simulink model "Perfect_Lineaer"  (R2017a)
settings: Solver=VariableStepAuto  StartTime=0.0  StopTime=17  FixedStep=0.01  RelTol=1e-3
values from neighbouring files (symbols this model uses):
  A = [-4.65E-06	0.0001701	-0.0002836	0	0	0	-2.56E-06	-7.97E-06	3.61E-06 ... (first row only)    [surfaces_setup_test.m]
  A0 = [-4.65E-06	0.0001701	-0.0002836	0	0	0	0	-1.43	0 ... (first row only)    [surfaces_setup_test.m]
  a0_s2345 = [0;0;0.05;0.05]    [HW5_4_surfaces.m]    (also in TEST_aerosetup.m; surfaces_setup_test.m)
  A_2345 = c_2345.*b_2345    [HW5_4_surfaces.m]    (also in TEST_aerosetup.m; surfaces_setup_test.m)
  Aileron_left = 0    [HW5_4_surfaces.m]    (also in TEST_aerosetup.m; surfaces_setup_test.m)
  Aileron_right = 0    [HW5_4_surfaces.m]    (also in TEST_aerosetup.m; surfaces_setup_test.m)
  B = [-7.98E-09	7.83E-09	1.68E-09	2.75E-10 ... (first row only)    [surfaces_setup_test.m]
  B0 = [-6.2	6.2	0	0.45 ... (first row only)    [surfaces_setup_test.m]
  c_2345 = [0.075;0.08;0.1;0.1]    [HW5_4_surfaces.m]    (also in TEST_aerosetup.m; surfaces_setup_test.m)
  CD0_s2345 = [0.01;0.01;0.01;0.01]    [HW5_4_surfaces.m]    (also in TEST_aerosetup.m; surfaces_setup_test.m)
  CDa_s2345 = [1;1;1;1]    [HW5_4_surfaces.m]    (also in TEST_aerosetup.m; surfaces_setup_test.m)
  CL0_2345 = [0;0; 0.05; 0.05]    [HW5_4_surfaces.m]    (also in TEST_aerosetup.m; surfaces_setup_test.m)
  CLa = 2*pi*(r./(2+r))    [HW5_4_surfaces.m]    (also in TEST_aerosetup.m; surfaces_setup_test.m)
  CM0_s2345 = [0;0;-0.05;-0.05]    [HW5_4_surfaces.m]    (also in TEST_aerosetup.m; surfaces_setup_test.m)
  CMa_s2345 = [0; 0; 0; 0]    [HW5_4_surfaces.m]    (also in TEST_aerosetup.m; surfaces_setup_test.m)
  e_s2345 = [0.8;0.8;0.9;0.9]    [HW5_4_surfaces.m]    (also in TEST_aerosetup.m; surfaces_setup_test.m)
  elevator = 0    [HW5_4_surfaces.m]    (also in TEST_aerosetup.m; surfaces_setup_test.m)
  Fext_N = -g_EN * m    [HW5_4_surfaces.m]    (also in TEST_aerosetup.m = [10 10 10]; surfaces_setup_test.m)
  g_EN = [0; 0; 9.81]    [HW5_4_surfaces.m]    (also in TEST_aerosetup.m = [0; 0; 9.8]; surfaces_setup_test.m)
  i_s2345 = [0; 0; 0.05; 0.05;]    [HW5_4_surfaces.m]    (also in TEST_aerosetup.m; surfaces_setup_test.m)
  J_cgp = ones(3)    [surfaces_setup_test.m]
  M_total = sum(MnG(:,1))/1000    [HW5_4_surfaces.m]    (also in TEST_aerosetup.m; surfaces_setup_test.m = sum(MnG1(:,1))/1000)
  Mext_B = [0; 0; 0]    [HW5_4_surfaces.m]    (also in TEST_aerosetup.m = [1; 1; 1]; surfaces_setup_test.m)
  p_E_BE_ini = p_E_BE_ini_deg .* [deg2rad; deg2rad; 1]    [HW5_4_surfaces.m]    (also in TEST_aerosetup.m; surfaces_setup_test.m)
  r = b_2345./c_2345    [HW5_4_surfaces.m]    (also in TEST_aerosetup.m; surfaces_setup_test.m)
  Rearth = 6371000    [HW5_4_surfaces.m]    (also in TEST_aerosetup.m; surfaces_setup_test.m)
  rudder = 0    [HW5_4_surfaces.m]    (also in TEST_aerosetup.m; surfaces_setup_test.m)
  Theta_ini = Theta_ini_deg * deg2rad    [HW5_4_surfaces.m]    (also in TEST_aerosetup.m; surfaces_setup_test.m)
  U0 = [Aileron_right;Aileron_left;elevator;rudder]    [surfaces_setup_test.m]
  v_N_AE = [0;0;0]    [HW5_4_surfaces.m]    (also in TEST_aerosetup.m; surfaces_setup_test.m)
  Vbbe_int = [10; 0; 0]    [HW5_4_surfaces.m]    (also in TEST_aerosetup.m; surfaces_setup_test.m = [5; 0; 0])
  w_B_BE_ini = [1e0; 1e-2; 1e-2]    [HW5_4_surfaces.m]    (also in TEST_aerosetup.m; surfaces_setup_test.m)
  X0 = [w_B_BE_ini;Theta_ini;Vbbe_int]    [surfaces_setup_test.m]
  xyz_s = [[-0.76 0 0.16];[-0.76 0 -0.09];[-0.23 0.44 0];[-0.23 -0.44 0];]    [HW5_4_surfaces.m]    (also in TEST_aerosetup.m; surfaces_setup_test.m)
undefined symbols (not defined in the file or in its folder): Discrete, Earth, K, Time, WGS84
libraries: simulink x83, aerolibfltsims x5, dspsrcs4 x4, simulink_extras x4, dspinverses x3, vrlib x2, sharedtransform x1, aerolibtransform2 x1, aerolibutil x1, sharedutil x1, ctrlSharedLib x1
(part 5 of 8)

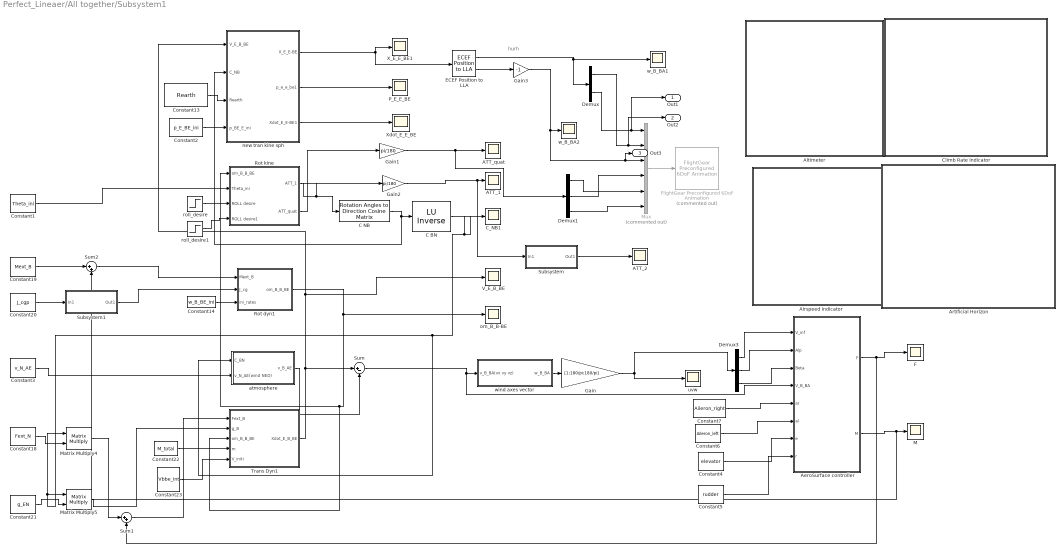
== system Perfect_Lineaer/All together/Subsystem1 ==
  note: hurh
  ATT_1 : Scope
  ATT_2 : Scope
  ATT_quat : Scope
  AeroSurface controller : Subsystem
  Airspeed Indicator : Subsystem  DialogController=aeroblksHMICreateDDGDialog  IsWebBlock=on  mask(MWDashboardBlock){webBlockId=e5e3171d-ff29-4451-bf74-d38876eec561, webBlockType=airspeedindicator, ShowInLibBrowser=on, ShowInitialText=on, HMISrcModelName=Perfect_Lineaer}
      mask prompts: webBlockId "WebBlock Id"; webBlockType "WebBlock Type"; HMISrcModelName "Source Model"
      mask help: aeroblksHMI:aeroblkhmi:AirspeedIndicatorDialogDesc
      mask Help: eval('asbhmihelp(''airspeedindicator'')');
      mask Display:
      | if strcmp(get_param(bdroot(gcb),'BlockDiagramType'), 'library')
      |  image([(matlabroot) '/toolbox/aeroblks/aeroblks/hmi/icons/AirspeedIndicatorIcon.svg'])
      | end
  Altimeter : Subsystem  DialogController=aeroblksHMICreateDDGDialog  IsWebBlock=on  mask(MWDashboardBlock){webBlockId=36990637-e96a-433a-956a-f44ed4ed9d1e, webBlockType=altimeter, ShowInLibBrowser=on, ShowInitialText=on, HMISrcModelName=Perfect_Lineaer}
      mask prompts: webBlockId "WebBlock Id"; webBlockType "WebBlock Type"; HMISrcModelName "Source Model"
      mask help: aeroblksHMI:aeroblkhmi:AltimeterDialogDesc
      mask Help: eval('asbhmihelp(''altimeter'')');
      mask Display:
      | if strcmp(get_param(bdroot(gcb),'BlockDiagramType'), 'library')
      |  image([(matlabroot) '/toolbox/aeroblks/aeroblks/hmi/icons/AltimeterIcon.svg'])
      | end
  Artificial Horizon : Subsystem  DialogController=aeroblksHMICreateDDGDialog  IsWebBlock=on  mask(MWDashboardBlock){webBlockId=4cd5d09c-38f7-433d-892c-50154f5485b8, webBlockType=artificialhorizon, ShowInLibBrowser=on, ShowInitialText=on, HMISrcModelName=Perfect_Lineaer}
      mask prompts: webBlockId "WebBlock Id"; webBlockType "WebBlock Type"; HMISrcModelName "Source Model"
      mask help: aeroblksHMI:aeroblkhmi:ArtificialHorizonDialogDesc
      mask Help: eval('asbhmihelp(''artificialhorizon'')');
      mask Display:
      | if strcmp(get_param(bdroot(gcb),'BlockDiagramType'), 'library')
      |  image([(matlabroot) '/toolbox/aeroblks/aeroblks/hmi/icons/ArtificialHorizonIcon.svg'])
      | end
  C BN : dspinverses/ LU Inverse
      settings: SourceProductName=DSP System Toolbox
  C NB : sharedtransform/Rotation Angles to Direction Cosine Matrix  rotationOrder=ZYX
  C_NB1 : Scope
  Climb Rate Indicator : Subsystem  DialogController=aeroblksHMICreateDDGDialog  IsWebBlock=on  mask(MWDashboardBlock){webBlockId=79e6d40e-4c73-4bf3-981b-23b4e158f69b, webBlockType=climbindicator, ShowInLibBrowser=on, ShowInitialText=on, HMISrcModelName=Perfect_Lineaer}
      mask prompts: webBlockId "WebBlock Id"; webBlockType "WebBlock Type"; HMISrcModelName "Source Model"
      mask help: aeroblksHMI:aeroblkhmi:ClimbIndicatorDialogDesc
      mask Help: eval('asbhmihelp(''climbindicator'')');
      mask Display:
      | if strcmp(get_param(bdroot(gcb),'BlockDiagramType'), 'library')
      |  image([(matlabroot) '/toolbox/aeroblks/aeroblks/hmi/icons/ClimbIndicatorIcon.svg'])
      | end
  Constant1 : Constant  Value=Theta_ini
  Constant13 : Constant  Value=Rearth
  Constant14 : Constant  Value=w_B_BE_ini
  Constant18 : Constant  Value=Fext_N
  Constant19 : Constant  Value=Mext_B
  Constant2 : Constant  Value=p_E_BE_ini  VectorParams1D=off
  Constant20 : Constant  Value=J_cgp
  Constant21 : Constant  Value=g_EN
  Constant22 : Constant  Value=M_total
  Constant23 : Constant  Value=Vbbe_int
  Constant3 : Constant  Value=v_N_AE
  Constant4 : Constant  Value=elevator
  Constant5 : Constant  Value=rudder
  Constant6 : Constant  Value=Aileron_left
  Constant7 : Constant  Value=Aileron_right
  Demux : Demux  Outputs=2
  Demux1 : Demux  Outputs=3
  Demux3 : Demux  Outputs=3
  ECEF Position to LLA : aerolibtransform2/ECEF Position to LLA  units=Metric (MKS)  ptype=Earth (WGS84)  F=1/298.257223563  R=6378137
      settings: SourceProductName=Aerospace Blockset  SourceProductBaseCode=AE
  F : Scope
  FlightGear Preconfigured 6DoF Animation : aerolibfltsims/FlightGear Preconfigured 6DoF Animation  Commented=on  xFlightGearVersion=v3.0  DestinationIpAddress=127.0.0.1  DestinationPort=5502  SampleTime=1/50
      settings: SourceProductName=Aerospace Blockset
  Gain : Gain  Gain=[1;180/pi;180/pi]
  Gain1 : Gain  Gain=pi/180
  Gain2 : Gain  Gain=pi/180
  Gain3 : Gain  Gain=-1
  M : Scope
  Matrix Multiply4 : Product  Multiplication=Matrix(*)
  Matrix Multiply5 : Product  Multiplication=Matrix(*)
  Mux : Mux  Commented=on  Inputs=6
  P_E_E_BE : Scope
  Rot dyn1 : Subsystem
  Rot kine : Subsystem
  Subsystem : Subsystem
  Subsystem1 : Subsystem
  Sum : Sum  Inputs=|+-
  Sum1 : Sum  Inputs=|++
  Sum2 : Sum  Inputs=|++
  Trans Dyn1 : Subsystem
  V_E_B_BE : Scope
  "X_E_E_BE1 " : Scope
  Xdot_E_E_BE : Scope
  atmosphere : Subsystem
  new tran kine sph : Subsystem
  om_B_B-BE : Scope
  roll_desire : Step  Time=0  After=0  SampleTime=0
  roll_desire1 : Step  Time=0  After=0  SampleTime=0
  uvw : Scope
  w_B_BA1 : Scope
  w_B_BA2 : Scope
  wind axes vector : Subsystem
  Out1 : Outport
  Out2 : Outport  Port=2
  Out3 : Outport  Port=3
  wires:
  Subsystem1/1(Out1) -> Rot dyn1/2(J_cg)
  Constant20/1 -> Subsystem1/1(In1)
  Sum1/1 -> Trans Dyn1/1(Fext_B)
  Gain3/1 -> w_B_BA2/1, Out3/1, Mux/3
  ECEF Position to LLA/1 -> Demux/1, w_B_BA1/1
  Constant19/1 -> Sum2/1
  roll_desire/1 -> Rot kine/3(ROLL desire)
  Matrix Multiply4/1 -> Sum1/1
  ECEF Position to LLA/2 -> Gain3/1
  Demux1/2 -> Mux/4
  Gain2/1 -> Subsystem/1(In1), ATT_1/1
  Rot kine/2(ATT_quat) -> Gain1/1
  AeroSurface controller/1(F) -> Sum1/2, F/1
  Demux3/1 -> AeroSurface controller/1(V_inf)
  Demux3/2 -> AeroSurface controller/2(Alp)
  Constant21/1 -> Matrix Multiply5/2
  Demux1/3 -> Mux/6
  C NB/1 -> new tran kine sph/2(C_NB), C BN/1
  Constant5/1 -> AeroSurface controller/8(r)
  Constant7/1 -> AeroSurface controller/5(ar)
  Rot dyn1/1(om_B_B_BE) -> Trans Dyn1/3(om_B_B_BE), Rot kine/1(om_B_B_BE), om_B_B-BE/1
  atmosphere/1(v_B_AE) -> Sum/2
  Sum/1 -> AeroSurface controller/4(V_B_BA), wind axes vector/1(v_B_BA(vx vy vz))
  Constant22/1 -> Trans Dyn1/4(m)
  Constant4/1 -> AeroSurface controller/7(e)
  Constant1/1 -> Rot kine/2(Theta_ini)
  Gain1/1 -> Demux1/1, ATT_quat/1
  Sum2/1 -> Rot dyn1/1(Mext_B)
  AeroSurface controller/2(M) -> Sum2/2, M/1
  Demux1/1 -> Mux/5
  Mux/1 -> FlightGear Preconfigured 6DoF Animation/1
  Constant13/1 -> new tran kine sph/3(Rearth)
  Constant14/1 -> Rot dyn1/3(ini_rates)
  roll_desire1/1 -> Rot kine/4(ROLL desire1)
  new tran kine sph/3(Xdot_E_E-BE1) -> Xdot_E_E_BE/1
  Rot kine/1(ATT_1) -> C NB/1, Gain2/1
  C BN/1 -> atmosphere/1(C_BN), Matrix Multiply5/1, Matrix Multiply4/1, C_NB1/1
  new tran kine sph/1(X_E_E-BE) -> ECEF Position to LLA/1, "X_E_E_BE1 "/1
  Subsystem/1(Out1) -> ATT_2/1
  Constant6/1 -> AeroSurface controller/6(al)
  Constant3/1 -> atmosphere/2(v_N_AE(wind NED))
  new tran kine sph/2(p_e_e_be1) -> P_E_E_BE/1
  Trans Dyn1/1(Xdot_E_B_BE) -> new tran kine sph/1(V_E_B_BE), V_E_B_BE/1, Sum/1
  Gain/1 -> Demux3/1, uvw/1
  Constant18/1 -> Matrix Multiply4/2
  wind axes vector/1(w_B_BA) -> Gain/1
  Constant23/1 -> Trans Dyn1/5(V_initi)
  Demux/1 -> Out2/1, Mux/2
  Demux/2 -> Out1/1, Mux/1
  Demux3/3 -> AeroSurface controller/3(Beta)
  Constant2/1 -> new tran kine sph/4(p_BE_E_ini)
  Matrix Multiply5/1 -> Trans Dyn1/2(g_B)

== system Perfect_Lineaer/All together/Subsystem2 ==
  note: State loop
  note: Inner loop
  Rudder : Inport
  Elevator : Inport  Port=2
  Aileron_left : Inport  Port=3
  A : Gain  Gain=A  Multiplication=Matrix(K*u)
  B : Gain  Gain=B  Multiplication=Matrix(K*u)
  Constant1 : Constant  Value=0
  Constant2 : Constant  Value=X0
  Demux : Demux  Outputs=9
  Integrator : Integrator  InitialConditionSource=external
  KD_Based on Rlocus : Gain
  Mux : Mux  Inputs=9
  Mux1 : Mux
  Scope : Scope
  Scope1 : Scope
  Sum : Sum  Inputs=|++
  Sum1 : Sum  Inputs=|++
  Sum4 : Sum  Inputs=|+-
  selector : Subsystem
  R(yaw) : Outport
  Q(pitch) : Outport  Port=2
  P(roll) : Outport  Port=3
  wires:
  Elevator/1 -> Mux1/3
  Sum1/1 -> Mux/8
  KD_Based on Rlocus/1 -> Sum1/2
  Demux/8 -> Sum1/1
  Rudder/1 -> Mux1/4
  Constant1/1 -> Mux1/1
  Mux1/1 -> B/1
  Mux/1 -> Sum4/1
  Demux/1 -> Mux/1
  Demux/5 -> Mux/5
  A/1 -> Sum/2
  Sum4/1 -> Sum/1
  Integrator/1 -> A/1, selector/1(In1), Scope/1, Sum4/2
  Demux/9 -> Mux/9
  Demux/4 -> Mux/4
  Demux/2 -> Mux/2
  B/1 -> Demux/1
  selector/1(Out1) -> KD_Based on Rlocus/1, Scope1/1
  Sum/1 -> Integrator/1
  Demux/3 -> Mux/3
  Constant2/1 -> Integrator/2
  Demux/6 -> Mux/6
  Demux/7 -> Mux/7
  selector/2(Out2) -> Q(pitch)/1
  selector/3(Out3) -> R(yaw)/1
  selector/4(Out4) -> P(roll)/1
  Aileron_left/1 -> Mux1/2

== system Perfect_Lineaer/All together/Subsystem5 ==
  note: State loop
  note: Inner loop
  Rudder : Inport
  Elevator : Inport  Port=2
  Aileron_left : Inport  Port=3
  A : Gain  Gain=A  Multiplication=Matrix(K*u)
  B : Gain  Gain=B  Multiplication=Matrix(K*u)
  Constant1 : Constant  Value=0
  Constant2 : Constant  Value=X0
  Demux : Demux  Outputs=9
  Integrator : Integrator  InitialConditionSource=external
  KD_Based on Rlocus : Gain
  Mux : Mux  Inputs=9
  Mux1 : Mux
  Scope : Scope
  Scope1 : Scope
  Sum : Sum  Inputs=|++
  Sum1 : Sum  Inputs=|++
  Sum4 : Sum  Inputs=|+-
  selector : Subsystem
  R(yaw) : Outport
  Q(pitch) : Outport  Port=2
  P(roll) : Outport  Port=3
  wires:
  Elevator/1 -> Mux1/3
  Sum1/1 -> Mux/8
  KD_Based on Rlocus/1 -> Sum1/2
  Demux/8 -> Sum1/1
  Rudder/1 -> Mux1/4
  Constant1/1 -> Mux1/1
  Mux1/1 -> B/1
  Mux/1 -> Sum4/1
  Demux/1 -> Mux/1
  Demux/5 -> Mux/5
  A/1 -> Sum/2
  Sum4/1 -> Sum/1
  Integrator/1 -> A/1, selector/1(In1), Scope/1, Sum4/2
  Demux/9 -> Mux/9
  Demux/4 -> Mux/4
  Demux/2 -> Mux/2
  B/1 -> Demux/1
  selector/1(Out1) -> KD_Based on Rlocus/1, Scope1/1
  Sum/1 -> Integrator/1
  Demux/3 -> Mux/3
  Constant2/1 -> Integrator/2
  Demux/6 -> Mux/6
  Demux/7 -> Mux/7
  selector/2(Out2) -> Q(pitch)/1
  selector/3(Out3) -> R(yaw)/1
  selector/4(Out4) -> P(roll)/1
  Aileron_left/1 -> Mux1/2

== system Perfect_Lineaer/All together/Turn Coordinator ==

== system Perfect_Lineaer/Command size/Subsystem ==
  note: State loop
  note: Inner loop
  Rudder : Inport
  A : Gain  Gain=A  Multiplication=Matrix(K*u)
  B : Gain  Gain=B  Multiplication=Matrix(K*u)
  Constant1 : Constant  Value=0
  Constant2 : Constant  Value=X0
  Demux : Demux  Outputs=9
  Integrator : Integrator  InitialConditionSource=external
  KD_Based on Rlocus : Gain
  Mux : Mux  Inputs=9
  Mux1 : Mux
  Scope : Scope
  Scope1 : Scope
  Sum : Sum  Inputs=|++
  Sum1 : Sum  Inputs=|++
  Sum4 : Sum  Inputs=|+-
  selector : Subsystem
  R(yaw) : Outport
  wires:
  Sum1/1 -> Mux/8
  KD_Based on Rlocus/1 -> Sum1/2
  Demux/8 -> Sum1/1
  selector/2(Out2) -> R(yaw)/1
  Rudder/1 -> Mux1/4
  Constant1/1 -> Mux1/1, Mux1/2, Mux1/3
  Mux1/1 -> B/1
  Mux/1 -> Sum4/1
  Demux/1 -> Mux/1
  Demux/5 -> Mux/5
  A/1 -> Sum/2
  Sum4/1 -> Sum/1
  Integrator/1 -> A/1, selector/1(In1), Scope/1, Sum4/2
  Demux/9 -> Mux/9
  Demux/4 -> Mux/4
  Demux/2 -> Mux/2
  B/1 -> Demux/1
  selector/1(Out1) -> KD_Based on Rlocus/1, Scope1/1
  Sum/1 -> Integrator/1
  Demux/3 -> Mux/3
  Constant2/1 -> Integrator/2
  Demux/6 -> Mux/6
  Demux/7 -> Mux/7

== system Perfect_Lineaer/Command size/Subsystem1 ==
  note: State loop
  note: Inner loop
  Elevator : Inport
  A : Gain  Gain=A  Multiplication=Matrix(K*u)
  B : Gain  Gain=B  Multiplication=Matrix(K*u)
  Constant1 : Constant  Value=0
  Constant2 : Constant  Value=X0
  Demux : Demux  Outputs=9
  Integrator : Integrator  InitialConditionSource=external
  KD_Based on Rlocus : Gain
  Mux : Mux  Inputs=9
  Mux1 : Mux
  Scope : Scope
  Scope1 : Scope
  Sum : Sum  Inputs=|++
  Sum1 : Sum  Inputs=|++
  Sum4 : Sum  Inputs=|+-
  selector : Subsystem
  Q(pitch) : Outport
  wires:
  Elevator/1 -> Mux1/3
  Sum1/1 -> Mux/8
  KD_Based on Rlocus/1 -> Sum1/2
  Demux/8 -> Sum1/1
  Constant1/1 -> Mux1/4, Mux1/1, Mux1/2
  Mux1/1 -> B/1
  Mux/1 -> Sum4/1
  Demux/1 -> Mux/1
  Demux/5 -> Mux/5
  A/1 -> Sum/2
  Sum4/1 -> Sum/1
  Integrator/1 -> A/1, Scope/1, Sum4/2, selector/1(In1)
  Demux/9 -> Mux/9
  Demux/4 -> Mux/4
  Demux/2 -> Mux/2
  B/1 -> Demux/1
  selector/1(Out1) -> KD_Based on Rlocus/1, Scope1/1
  Sum/1 -> Integrator/1
  Demux/3 -> Mux/3
  Constant2/1 -> Integrator/2
  Demux/6 -> Mux/6
  Demux/7 -> Mux/7
  selector/2(Out2) -> Q(pitch)/1

== system Perfect_Lineaer/Command size/Subsystem2 ==
  note: State loop
  note: Inner loop
  Rudder : Inport
  A : Gain  Gain=A  Multiplication=Matrix(K*u)
  B : Gain  Gain=B  Multiplication=Matrix(K*u)
  Constant1 : Constant  Value=0
  Constant2 : Constant  Value=X0
  Demux : Demux  Outputs=9
  Integrator : Integrator  InitialConditionSource=external
  KD_Based on Rlocus : Gain
  Mux : Mux  Inputs=9
  Mux1 : Mux
  Scope : Scope
  Scope1 : Scope
  Sum : Sum  Inputs=|++
  Sum1 : Sum  Inputs=|++
  Sum4 : Sum  Inputs=|+-
  selector : Subsystem
  R(yaw) : Outport
  wires:
  Sum1/1 -> Mux/8
  KD_Based on Rlocus/1 -> Sum1/2
  Demux/8 -> Sum1/1
  selector/2(Out2) -> R(yaw)/1
  Rudder/1 -> Mux1/4
  Constant1/1 -> Mux1/1, Mux1/2, Mux1/3
  Mux1/1 -> B/1
  Mux/1 -> Sum4/1
  Demux/1 -> Mux/1
  Demux/5 -> Mux/5
  A/1 -> Sum/2
  Sum4/1 -> Sum/1
  Integrator/1 -> A/1, selector/1(In1), Scope/1, Sum4/2
  Demux/9 -> Mux/9
  Demux/4 -> Mux/4
  Demux/2 -> Mux/2
  B/1 -> Demux/1
  selector/1(Out1) -> KD_Based on Rlocus/1, Scope1/1
  Sum/1 -> Integrator/1
  Demux/3 -> Mux/3
  Constant2/1 -> Integrator/2
  Demux/6 -> Mux/6
  Demux/7 -> Mux/7

== system Perfect_Lineaer/Command size/Subsystem3 ==
  note: State loop
  note: Inner loop
  Elevator : Inport
  A : Gain  Gain=A  Multiplication=Matrix(K*u)
  B : Gain  Gain=B  Multiplication=Matrix(K*u)
  Constant1 : Constant  Value=0
  Constant2 : Constant  Value=X0
  Demux : Demux  Outputs=9
  Integrator : Integrator  InitialConditionSource=external
  KD_Based on Rlocus : Gain
  Mux : Mux  Inputs=9
  Mux1 : Mux
  Scope : Scope
  Scope1 : Scope
  Sum : Sum  Inputs=|++
  Sum1 : Sum  Inputs=|++
  Sum4 : Sum  Inputs=|+-
  selector : Subsystem
  Q(pitch) : Outport
  wires:
  Elevator/1 -> Mux1/3
  Sum1/1 -> Mux/8
  KD_Based on Rlocus/1 -> Sum1/2
  Demux/8 -> Sum1/1
  Constant1/1 -> Mux1/4, Mux1/1, Mux1/2
  Mux1/1 -> B/1
  Mux/1 -> Sum4/1
  Demux/1 -> Mux/1
  Demux/5 -> Mux/5
  A/1 -> Sum/2
  Sum4/1 -> Sum/1
  Integrator/1 -> A/1, Scope/1, Sum4/2, selector/1(In1)
  Demux/9 -> Mux/9
  Demux/4 -> Mux/4
  Demux/2 -> Mux/2
  B/1 -> Demux/1
  selector/1(Out1) -> KD_Based on Rlocus/1, Scope1/1
  Sum/1 -> Integrator/1
  Demux/3 -> Mux/3
  Constant2/1 -> Integrator/2
  Demux/6 -> Mux/6
  Demux/7 -> Mux/7
  selector/2(Out2) -> Q(pitch)/1

== system Perfect_Lineaer/Command size/Subsystem4 ==
  note: State loop
  note: Inner loop
  Aileron_r : Inport
  Aileron_l : Inport  Port=2
  A : Gain  Gain=A  Multiplication=Matrix(K*u)
  B : Gain  Gain=B  Multiplication=Matrix(K*u)
  Constant1 : Constant  Value=0
  Constant2 : Constant  Value=X0
  Demux : Demux  Outputs=9
  Integrator : Integrator  InitialConditionSource=external
  KD_Based on Rlocus : Gain
  Mux : Mux  Inputs=9
  Mux1 : Mux
  Scope : Scope
  Scope1 : Scope
  Sum : Sum  Inputs=|++
  Sum1 : Sum  Inputs=|++
  Sum4 : Sum  Inputs=|+-
  selector : Subsystem
  P(roll) : Outport
  wires:
  Aileron_r/1 -> Mux1/1
  Aileron_l/1 -> Mux1/2
  Sum1/1 -> Mux/8
  KD_Based on Rlocus/1 -> Sum1/2
  Demux/8 -> Sum1/1
  selector/2(Out2) -> P(roll)/1
  Constant1/1 -> Mux1/4, Mux1/3
  Mux1/1 -> B/1
  Mux/1 -> Sum4/1
  Demux/1 -> Mux/1
  Demux/5 -> Mux/5
  A/1 -> Sum/2
  Sum4/1 -> Sum/1
  Integrator/1 -> A/1, selector/1(In1), Scope/1, Sum4/2
  Demux/9 -> Mux/9
  Demux/4 -> Mux/4
  Demux/2 -> Mux/2
  B/1 -> Demux/1
  selector/1(Out1) -> KD_Based on Rlocus/1, Scope1/1
  Sum/1 -> Integrator/1
  Demux/3 -> Mux/3
  Constant2/1 -> Integrator/2
  Demux/6 -> Mux/6
  Demux/7 -> Mux/7

== system Perfect_Lineaer/Command size/Subsystem9 ==
  note: State loop
  note: Inner loop
  Aileron_r : Inport
  Aileron_l : Inport  Port=2
  A : Gain  Gain=A  Multiplication=Matrix(K*u)
  B : Gain  Gain=B  Multiplication=Matrix(K*u)
  Constant1 : Constant  Value=0
  Constant2 : Constant  Value=X0
  Demux : Demux  Outputs=9
  Integrator : Integrator  InitialConditionSource=external
  KD_Based on Rlocus : Gain
  Mux : Mux  Inputs=9
  Mux1 : Mux
  Scope : Scope
  Scope1 : Scope
  Sum : Sum  Inputs=|++
  Sum1 : Sum  Inputs=|++
  Sum4 : Sum  Inputs=|+-
  selector : Subsystem
  P(roll) : Outport
  wires:
  Aileron_r/1 -> Mux1/1
  Aileron_l/1 -> Mux1/2
  Sum1/1 -> Mux/8
  KD_Based on Rlocus/1 -> Sum1/2
  Demux/8 -> Sum1/1
  selector/2(Out2) -> P(roll)/1
  Constant1/1 -> Mux1/4, Mux1/3
  Mux1/1 -> B/1
  Mux/1 -> Sum4/1
  Demux/1 -> Mux/1
  Demux/5 -> Mux/5
  A/1 -> Sum/2
  Sum4/1 -> Sum/1
  Integrator/1 -> A/1, selector/1(In1), Scope/1, Sum4/2
  Demux/9 -> Mux/9
  Demux/4 -> Mux/4
  Demux/2 -> Mux/2
  B/1 -> Demux/1
  selector/1(Out1) -> KD_Based on Rlocus/1, Scope1/1
  Sum/1 -> Integrator/1
  Demux/3 -> Mux/3
  Constant2/1 -> Integrator/2
  Demux/6 -> Mux/6
  Demux/7 -> Mux/7

== system Perfect_Lineaer/Decoupled/Artificial Horizon ==

== system Perfect_Lineaer/Decoupled/Heading Indicator ==

== system Perfect_Lineaer/Decoupled/Subsystem ==
  note: State loop
  note: Inner loop
  Rudder : Inport
  A : Gain  Gain=A  Multiplication=Matrix(K*u)
  B : Gain  Gain=B  Multiplication=Matrix(K*u)
  Constant1 : Constant  Value=0
  Constant2 : Constant  Value=X0
  Demux : Demux  Outputs=9
  Integrator : Integrator  InitialConditionSource=external
  KD_Based on Rlocus : Gain
  Mux : Mux  Inputs=9
  Mux1 : Mux
  Scope : Scope
  Scope1 : Scope
  Sum : Sum  Inputs=|++
  Sum1 : Sum  Inputs=|++
  Sum4 : Sum  Inputs=|+-
  selector : Subsystem
  R(yaw) : Outport
  wires:
  Sum1/1 -> Mux/8
  KD_Based on Rlocus/1 -> Sum1/2
  Demux/8 -> Sum1/1
  selector/2(Out2) -> R(yaw)/1
  Rudder/1 -> Mux1/4
  Constant1/1 -> Mux1/1, Mux1/2, Mux1/3
  Mux1/1 -> B/1
  Mux/1 -> Sum4/1
  Demux/1 -> Mux/1
  Demux/5 -> Mux/5
  A/1 -> Sum/2
  Sum4/1 -> Sum/1
  Integrator/1 -> A/1, selector/1(In1), Scope/1, Sum4/2
  Demux/9 -> Mux/9
  Demux/4 -> Mux/4
  Demux/2 -> Mux/2
  B/1 -> Demux/1
  selector/1(Out1) -> KD_Based on Rlocus/1, Scope1/1
  Sum/1 -> Integrator/1
  Demux/3 -> Mux/3
  Constant2/1 -> Integrator/2
  Demux/6 -> Mux/6
  Demux/7 -> Mux/7

== system Perfect_Lineaer/Decoupled/Subsystem1 ==
  note: State loop
  note: Inner loop
  Elevator : Inport
  A : Gain  Gain=A  Multiplication=Matrix(K*u)
  B : Gain  Gain=B  Multiplication=Matrix(K*u)
  Constant1 : Constant  Value=0
  Constant2 : Constant  Value=X0
  Demux : Demux  Outputs=9
  Integrator : Integrator  InitialConditionSource=external
  KD_Based on Rlocus : Gain
  Mux : Mux  Inputs=9
  Mux1 : Mux
  Scope : Scope
  Scope1 : Scope
  Sum : Sum  Inputs=|++
  Sum1 : Sum  Inputs=|++
  Sum4 : Sum  Inputs=|+-
  selector : Subsystem
  Q(pitch) : Outport
  wires:
  Elevator/1 -> Mux1/3
  Sum1/1 -> Mux/8
  KD_Based on Rlocus/1 -> Sum1/2
  Demux/8 -> Sum1/1
  Constant1/1 -> Mux1/4, Mux1/1, Mux1/2
  Mux1/1 -> B/1
  Mux/1 -> Sum4/1
  Demux/1 -> Mux/1
  Demux/5 -> Mux/5
  A/1 -> Sum/2
  Sum4/1 -> Sum/1
  Integrator/1 -> A/1, Scope/1, Sum4/2, selector/1(In1)
  Demux/9 -> Mux/9
  Demux/4 -> Mux/4
  Demux/2 -> Mux/2
  B/1 -> Demux/1
  selector/1(Out1) -> KD_Based on Rlocus/1, Scope1/1
  Sum/1 -> Integrator/1
  Demux/3 -> Mux/3
  Constant2/1 -> Integrator/2
  Demux/6 -> Mux/6
  Demux/7 -> Mux/7
  selector/2(Out2) -> Q(pitch)/1

== system Perfect_Lineaer/Decoupled/Subsystem5 ==
  note: State loop
  note: Inner loop
  Rudder : Inport
  Elevator : Inport  Port=2
  A : Gain  Gain=A  Multiplication=Matrix(K*u)
  B : Gain  Gain=B  Multiplication=Matrix(K*u)
  Constant1 : Constant  Value=0
  Constant2 : Constant  Value=X0
  Demux : Demux  Outputs=9
  Integrator : Integrator  InitialConditionSource=external
  KD_Based on Rlocus : Gain
  Mux : Mux  Inputs=9
  Mux1 : Mux
  Scope : Scope
  Scope1 : Scope
  Sum : Sum  Inputs=|++
  Sum1 : Sum  Inputs=|++
  Sum4 : Sum  Inputs=|+-
  selector : Subsystem
  R(yaw) : Outport
  Q(pitch) : Outport  Port=2
  wires:
  Elevator/1 -> Mux1/3
  Sum1/1 -> Mux/8
  KD_Based on Rlocus/1 -> Sum1/2
  Demux/8 -> Sum1/1
  Rudder/1 -> Mux1/4
  Constant1/1 -> Mux1/1, Mux1/2
  Mux1/1 -> B/1
  Mux/1 -> Sum4/1
  Demux/1 -> Mux/1
  Demux/5 -> Mux/5
  A/1 -> Sum/2
  Sum4/1 -> Sum/1
  Integrator/1 -> A/1, selector/1(In1), Scope/1, Sum4/2
  Demux/9 -> Mux/9
  Demux/4 -> Mux/4
  Demux/2 -> Mux/2
  B/1 -> Demux/1
  selector/1(Out1) -> KD_Based on Rlocus/1, Scope1/1
  Sum/1 -> Integrator/1
  Demux/3 -> Mux/3
  Constant2/1 -> Integrator/2
  Demux/6 -> Mux/6
  Demux/7 -> Mux/7
  selector/2(Out2) -> Q(pitch)/1
  selector/3(Out3) -> R(yaw)/1

== system Perfect_Lineaer/Decoupled/Subsystem9 ==
  note: State loop
  note: Inner loop
  Aileron_r : Inport
  Aileron_l : Inport  Port=2
  A : Gain  Gain=A  Multiplication=Matrix(K*u)
  B : Gain  Gain=B  Multiplication=Matrix(K*u)
  Constant1 : Constant  Value=0
  Constant2 : Constant  Value=X0
  Demux : Demux  Outputs=9
  Integrator : Integrator  InitialConditionSource=external
  KD_Based on Rlocus : Gain
  Mux : Mux  Inputs=9
  Mux1 : Mux
  Scope : Scope
  Scope1 : Scope
  Sum : Sum  Inputs=|++
  Sum1 : Sum  Inputs=|++
  Sum4 : Sum  Inputs=|+-
  selector : Subsystem
  P(roll) : Outport
  wires:
  Aileron_r/1 -> Mux1/1
  Aileron_l/1 -> Mux1/2
  Sum1/1 -> Mux/8
  KD_Based on Rlocus/1 -> Sum1/2
  Demux/8 -> Sum1/1
  selector/2(Out2) -> P(roll)/1
  Constant1/1 -> Mux1/4, Mux1/3
  Mux1/1 -> B/1
  Mux/1 -> Sum4/1
  Demux/1 -> Mux/1
  Demux/5 -> Mux/5
  A/1 -> Sum/2
  Sum4/1 -> Sum/1
  Integrator/1 -> A/1, selector/1(In1), Scope/1, Sum4/2
  Demux/9 -> Mux/9
  Demux/4 -> Mux/4
  Demux/2 -> Mux/2
  B/1 -> Demux/1
  selector/1(Out1) -> KD_Based on Rlocus/1, Scope1/1
  Sum/1 -> Integrator/1
  Demux/3 -> Mux/3
  Constant2/1 -> Integrator/2
  Demux/6 -> Mux/6
  Demux/7 -> Mux/7

== system Perfect_Lineaer/Decoupled/Turn Coordinator ==

== system Perfect_Lineaer/Pilot command(STT)/Linearized system ==
  Commands : Inport
  States : Outport
  wires:
  Commands/1 -> States/1

== system Perfect_Lineaer/Pilot command(STT)/Sensor(s) ==
  Input : Inport
  Noise : Inport  Port=2
  Scope2 : Scope
  output : Outport
  wires:
  Input/1 -> output/1
  Noise/1 -> Scope2/1

== system Perfect_Lineaer/Pilot command(STT)/Subsystem ==
  note: State loop
  note: Inner loop
  Rudder : Inport
  A : Gain  Gain=A  Multiplication=Matrix(K*u)
  B : Gain  Gain=B  Multiplication=Matrix(K*u)
  Constant1 : Constant  Value=0
  Constant2 : Constant  Value=X0
  Demux : Demux  Outputs=9
  Integrator : Integrator  InitialConditionSource=external
  KD_Based on Rlocus : Gain
  Mux : Mux  Inputs=9
  Mux1 : Mux
  Scope : Scope
  Scope1 : Scope
  Sum : Sum  Inputs=|++
  Sum1 : Sum  Inputs=|++
  Sum4 : Sum  Inputs=|+-
  selector : Subsystem
  R(yaw) : Outport
  wires:
  Sum1/1 -> Mux/8
  KD_Based on Rlocus/1 -> Sum1/2
  Demux/8 -> Sum1/1
  selector/2(Out2) -> R(yaw)/1
  Rudder/1 -> Mux1/4
  Constant1/1 -> Mux1/1, Mux1/2, Mux1/3
  Mux1/1 -> B/1
  Mux/1 -> Sum4/1
  Demux/1 -> Mux/1
  Demux/5 -> Mux/5
  A/1 -> Sum/2
  Sum4/1 -> Sum/1
  Integrator/1 -> A/1, selector/1(In1), Scope/1, Sum4/2
  Demux/9 -> Mux/9
  Demux/4 -> Mux/4
  Demux/2 -> Mux/2
  B/1 -> Demux/1
  selector/1(Out1) -> KD_Based on Rlocus/1, Scope1/1
  Sum/1 -> Integrator/1
  Demux/3 -> Mux/3
  Constant2/1 -> Integrator/2
  Demux/6 -> Mux/6
  Demux/7 -> Mux/7

== system Perfect_Lineaer/Pilot command(STT)/Subsystem1 ==
  note: State loop
  note: Inner loop
  Elevator : Inport
  A : Gain  Gain=A  Multiplication=Matrix(K*u)
  B : Gain  Gain=B  Multiplication=Matrix(K*u)
  Constant1 : Constant  Value=0
  Constant2 : Constant  Value=X0
  Demux : Demux  Outputs=9
  Integrator : Integrator  InitialConditionSource=external
  KD_Based on Rlocus : Gain
  Mux : Mux  Inputs=9
  Mux1 : Mux
  Scope : Scope
  Scope1 : Scope
  Sum : Sum  Inputs=|++
  Sum1 : Sum  Inputs=|++
  Sum4 : Sum  Inputs=|+-
  selector : Subsystem
  Q(pitch) : Outport
  wires:
  Elevator/1 -> Mux1/3
  Sum1/1 -> Mux/8
  KD_Based on Rlocus/1 -> Sum1/2
  Demux/8 -> Sum1/1
  Constant1/1 -> Mux1/4, Mux1/1, Mux1/2
  Mux1/1 -> B/1
  Mux/1 -> Sum4/1
  Demux/1 -> Mux/1
  Demux/5 -> Mux/5
  A/1 -> Sum/2
  Sum4/1 -> Sum/1
  Integrator/1 -> A/1, Scope/1, Sum4/2, selector/1(In1)
  Demux/9 -> Mux/9
  Demux/4 -> Mux/4
  Demux/2 -> Mux/2
  B/1 -> Demux/1
  selector/1(Out1) -> KD_Based on Rlocus/1, Scope1/1
  Sum/1 -> Integrator/1
  Demux/3 -> Mux/3
  Constant2/1 -> Integrator/2
  Demux/6 -> Mux/6
  Demux/7 -> Mux/7
  selector/2(Out2) -> Q(pitch)/1

== system Perfect_Lineaer/Pilot command(STT)/Subsystem5 ==
  note: State loop
  note: Inner loop
  Rudder : Inport
  Elevator : Inport  Port=2
  A : Gain  Gain=A  Multiplication=Matrix(K*u)
  B : Gain  Gain=B  Multiplication=Matrix(K*u)
  Constant1 : Constant  Value=0
  Constant2 : Constant  Value=X0
  Demux : Demux  Outputs=9
  Integrator : Integrator  InitialConditionSource=external
  KD_Based on Rlocus : Gain
  Mux : Mux  Inputs=9
  Mux1 : Mux
  Scope : Scope
  Scope1 : Scope
  Sum : Sum  Inputs=|++
  Sum1 : Sum  Inputs=|++
  Sum4 : Sum  Inputs=|+-
  selector : Subsystem
  R(yaw) : Outport
  Q(pitch) : Outport  Port=2
  wires:
  Elevator/1 -> Mux1/3
  Sum1/1 -> Mux/8
  KD_Based on Rlocus/1 -> Sum1/2
  Demux/8 -> Sum1/1
  Rudder/1 -> Mux1/4
  Constant1/1 -> Mux1/1, Mux1/2
  Mux1/1 -> B/1
  Mux/1 -> Sum4/1
  Demux/1 -> Mux/1
  Demux/5 -> Mux/5
  A/1 -> Sum/2
  Sum4/1 -> Sum/1
  Integrator/1 -> A/1, selector/1(In1), Scope/1, Sum4/2
  Demux/9 -> Mux/9
  Demux/4 -> Mux/4
  Demux/2 -> Mux/2
  B/1 -> Demux/1
  selector/1(Out1) -> KD_Based on Rlocus/1, Scope1/1
  Sum/1 -> Integrator/1
  Demux/3 -> Mux/3
  Constant2/1 -> Integrator/2
  Demux/6 -> Mux/6
  Demux/7 -> Mux/7
  selector/2(Out2) -> Q(pitch)/1
  selector/3(Out3) -> R(yaw)/1

== system Perfect_Lineaer/Really skid to turn/Artificial Horizon ==

== system Perfect_Lineaer/Really skid to turn/Heading Indicator ==

== system Perfect_Lineaer/Really skid to turn/Subsystem5 ==
  note: State loop
  note: Inner loop
  Rudder : Inport
  Elevator : Inport  Port=2
  A : Gain  Gain=A  Multiplication=Matrix(K*u)
  B : Gain  Gain=B  Multiplication=Matrix(K*u)
  Constant1 : Constant  Value=0
  Constant2 : Constant  Value=X0
  Demux : Demux  Outputs=9
  Integrator : Integrator  InitialConditionSource=external
  KD_Based on Rlocus : Gain
  Mux : Mux  Inputs=9
  Mux1 : Mux
  Scope : Scope
  Scope1 : Scope
  Sum : Sum  Inputs=|++
  Sum1 : Sum  Inputs=|++
  Sum4 : Sum  Inputs=|+-
  selector : Subsystem
  R(yaw) : Outport
  Q(pitch) : Outport  Port=2
  wires:
  Elevator/1 -> Mux1/3
  Sum1/1 -> Mux/8
  KD_Based on Rlocus/1 -> Sum1/2
  Demux/8 -> Sum1/1
  Rudder/1 -> Mux1/4
  Constant1/1 -> Mux1/1, Mux1/2
  Mux1/1 -> B/1
  Mux/1 -> Sum4/1
  Demux/1 -> Mux/1
  Demux/5 -> Mux/5
  A/1 -> Sum/2
  Sum4/1 -> Sum/1
  Integrator/1 -> A/1, selector/1(In1), Scope/1, Sum4/2
  Demux/9 -> Mux/9
  Demux/4 -> Mux/4
  Demux/2 -> Mux/2
  B/1 -> Demux/1
  selector/1(Out1) -> KD_Based on Rlocus/1, Scope1/1
  Sum/1 -> Integrator/1
  Demux/3 -> Mux/3
  Constant2/1 -> Integrator/2
  Demux/6 -> Mux/6
  Demux/7 -> Mux/7
  selector/2(Out2) -> Q(pitch)/1
  selector/3(Out3) -> R(yaw)/1

== system Perfect_Lineaer/Really skid to turn/Subsystem8 ==
  note: State loop
  note: Inner loop
  Aileron_r : Inport
  Aileron_l : Inport  Port=2
  A : Gain  Gain=A  Multiplication=Matrix(K*u)
  B : Gain  Gain=B  Multiplication=Matrix(K*u)
  Constant1 : Constant  Value=0
  Constant2 : Constant  Value=X0
  Demux : Demux  Outputs=9
  Integrator : Integrator  InitialConditionSource=external
  KD_Based on Rlocus : Gain
  Mux : Mux  Inputs=9
  Mux1 : Mux
  Scope : Scope
  Scope1 : Scope
  Sum : Sum  Inputs=|++
  Sum1 : Sum  Inputs=|++
  Sum4 : Sum  Inputs=|+-
  selector : Subsystem
  P(roll) : Outport
  wires:
  Aileron_l/1 -> Mux1/2
  Aileron_r/1 -> Mux1/1
  Sum1/1 -> Mux/8
  KD_Based on Rlocus/1 -> Sum1/2
  Demux/8 -> Sum1/1
  selector/2(Out2) -> P(roll)/1
  Constant1/1 -> Mux1/4, Mux1/3
  Mux1/1 -> B/1
  Mux/1 -> Sum4/1
  Demux/1 -> Mux/1
  Demux/5 -> Mux/5
  A/1 -> Sum/2
  Sum4/1 -> Sum/1
  Integrator/1 -> A/1, selector/1(In1), Scope/1, Sum4/2
  Demux/9 -> Mux/9
  Demux/4 -> Mux/4
  Demux/2 -> Mux/2
  B/1 -> Demux/1
  selector/1(Out1) -> KD_Based on Rlocus/1, Scope1/1
  Sum/1 -> Integrator/1
  Demux/3 -> Mux/3
  Constant2/1 -> Integrator/2
  Demux/6 -> Mux/6
  Demux/7 -> Mux/7

== system Perfect_Lineaer/Really skid to turn/Subsystem9 ==
  note: State loop
  note: Inner loop
  Aileron_r : Inport
  Aileron_l : Inport  Port=2
  A : Gain  Gain=A  Multiplication=Matrix(K*u)
  B : Gain  Gain=B  Multiplication=Matrix(K*u)
  Constant1 : Constant  Value=0
  Constant2 : Constant  Value=X0
  Demux : Demux  Outputs=9
  Integrator : Integrator  InitialConditionSource=external
  KD_Based on Rlocus : Gain
  Mux : Mux  Inputs=9
  Mux1 : Mux
  Scope : Scope
  Scope1 : Scope
  Sum : Sum  Inputs=|++
  Sum1 : Sum  Inputs=|++
  Sum4 : Sum  Inputs=|+-
  selector : Subsystem
  P(roll) : Outport
  wires:
  Aileron_r/1 -> Mux1/1
  Aileron_l/1 -> Mux1/2
  Sum1/1 -> Mux/8
  KD_Based on Rlocus/1 -> Sum1/2
  Demux/8 -> Sum1/1
  selector/2(Out2) -> P(roll)/1
  Constant1/1 -> Mux1/4, Mux1/3
  Mux1/1 -> B/1
  Mux/1 -> Sum4/1
  Demux/1 -> Mux/1
  Demux/5 -> Mux/5
  A/1 -> Sum/2
  Sum4/1 -> Sum/1
  Integrator/1 -> A/1, selector/1(In1), Scope/1, Sum4/2
  Demux/9 -> Mux/9
  Demux/4 -> Mux/4
  Demux/2 -> Mux/2
  B/1 -> Demux/1
  selector/1(Out1) -> KD_Based on Rlocus/1, Scope1/1
  Sum/1 -> Integrator/1
  Demux/3 -> Mux/3
  Constant2/1 -> Integrator/2
  Demux/6 -> Mux/6
  Demux/7 -> Mux/7

== system Perfect_Lineaer/Really skid to turn/Turn Coordinator ==

== system Perfect_Lineaer/Skid to turn (Lateral Dynamics don't change!)/Subsystem ==
  note: Inner loop
  note: State loop
  Rudder : Inport
  A : Gain  Gain=A  Multiplication=Matrix(K*u)
  B : Gain  Gain=B  Multiplication=Matrix(K*u)
  Constant1 : Constant  Value=0
  Constant2 : Constant  Value=X0
  Demux : Demux  Outputs=9
  Integrator : Integrator  InitialConditionSource=external
  KD_Based on Rlocus : Gain
  Mux : Mux  Inputs=9
  Mux1 : Mux
  Scope : Scope
  Scope1 : Scope
  Sum : Sum  Inputs=|++
  Sum1 : Sum  Inputs=|++
  Sum4 : Sum  Inputs=|+-
  selector : Subsystem
  R(yaw) : Outport
  wires:
  Demux/7 -> Mux/7
  Demux/6 -> Mux/6
  Constant2/1 -> Integrator/2
  Demux/3 -> Mux/3
  Sum/1 -> Integrator/1
  selector/1(Out1) -> Scope1/1, KD_Based on Rlocus/1
  B/1 -> Demux/1
  Demux/2 -> Mux/2
  Demux/4 -> Mux/4
  Demux/9 -> Mux/9
  Integrator/1 -> selector/1(In1), Sum4/2, Scope/1, A/1
  Sum4/1 -> Sum/1
  A/1 -> Sum/2
  Demux/5 -> Mux/5
  Demux/1 -> Mux/1
  Mux/1 -> Sum4/1
  Mux1/1 -> B/1
  Constant1/1 -> Mux1/3, Mux1/2, Mux1/1
  Rudder/1 -> Mux1/4
  selector/2(Out2) -> R(yaw)/1
  Demux/8 -> Sum1/1
  KD_Based on Rlocus/1 -> Sum1/2
  Sum1/1 -> Mux/8

== system Perfect_Lineaer/Skid to turn (Lateral Dynamics don't change!)/Subsystem1 ==
  note: Inner loop
  note: State loop
  Elevator : Inport
  A : Gain  Gain=A  Multiplication=Matrix(K*u)
  B : Gain  Gain=B  Multiplication=Matrix(K*u)
  Constant1 : Constant  Value=0
  Constant2 : Constant  Value=X0
  Demux : Demux  Outputs=9
  Integrator : Integrator  InitialConditionSource=external
  KD_Based on Rlocus : Gain
  Mux : Mux  Inputs=9
  Mux1 : Mux
  Scope : Scope
  Scope1 : Scope
  Sum : Sum  Inputs=|++
  Sum1 : Sum  Inputs=|++
  Sum4 : Sum  Inputs=|+-
  selector : Subsystem
  Q(pitch) : Outport
  wires:
  Demux/7 -> Mux/7
  Demux/6 -> Mux/6
  Constant2/1 -> Integrator/2
  Demux/3 -> Mux/3
  Sum/1 -> Integrator/1
  selector/1(Out1) -> Scope1/1, KD_Based on Rlocus/1
  B/1 -> Demux/1
  Demux/2 -> Mux/2
  Demux/4 -> Mux/4
  Demux/9 -> Mux/9
  Integrator/1 -> selector/1(In1), Sum4/2, Scope/1, A/1
  Sum4/1 -> Sum/1
  A/1 -> Sum/2
  Demux/5 -> Mux/5
  Demux/1 -> Mux/1
  Mux/1 -> Sum4/1
  Mux1/1 -> B/1
  Constant1/1 -> Mux1/2, Mux1/1, Mux1/4
  selector/2(Out2) -> Q(pitch)/1
  Demux/8 -> Sum1/1
  KD_Based on Rlocus/1 -> Sum1/2
  Sum1/1 -> Mux/8
  Elevator/1 -> Mux1/3

== system Perfect_Lineaer/Skid to turn (Lateral Dynamics don't change!)/Subsystem2 ==
  note: Inner loop
  note: State loop
  Rudder : Inport
  A : Gain  Gain=A  Multiplication=Matrix(K*u)
  B : Gain  Gain=B  Multiplication=Matrix(K*u)
  Constant1 : Constant  Value=0
  Constant2 : Constant  Value=X0
  Demux : Demux  Outputs=9
  Integrator : Integrator  InitialConditionSource=external
  KD_Based on Rlocus : Gain
  Mux : Mux  Inputs=9
  Mux1 : Mux
  Scope : Scope
  Scope1 : Scope
  Sum : Sum  Inputs=|++
  Sum1 : Sum  Inputs=|++
  Sum4 : Sum  Inputs=|+-
  selector : Subsystem
  R(yaw) : Outport
  wires:
  Demux/7 -> Mux/7
  Demux/6 -> Mux/6
  Constant2/1 -> Integrator/2
  Demux/3 -> Mux/3
  Sum/1 -> Integrator/1
  selector/1(Out1) -> Scope1/1, KD_Based on Rlocus/1
  B/1 -> Demux/1
  Demux/2 -> Mux/2
  Demux/4 -> Mux/4
  Demux/9 -> Mux/9
  Integrator/1 -> selector/1(In1), Sum4/2, Scope/1, A/1
  Sum4/1 -> Sum/1
  A/1 -> Sum/2
  Demux/5 -> Mux/5
  Demux/1 -> Mux/1
  Mux/1 -> Sum4/1
  Mux1/1 -> B/1
  Constant1/1 -> Mux1/3, Mux1/2, Mux1/1
  Rudder/1 -> Mux1/4
  selector/2(Out2) -> R(yaw)/1
  Demux/8 -> Sum1/1
  KD_Based on Rlocus/1 -> Sum1/2
  Sum1/1 -> Mux/8

== system Perfect_Lineaer/Skid to turn (Lateral Dynamics don't change!)/Subsystem3 ==
  note: Inner loop
  note: State loop
  Rudder : Inport
  A : Gain  Gain=A  Multiplication=Matrix(K*u)
  B : Gain  Gain=B  Multiplication=Matrix(K*u)
  Constant1 : Constant  Value=0
  Constant2 : Constant  Value=X0
  Demux : Demux  Outputs=9
  Integrator : Integrator  InitialConditionSource=external
  KD_Based on Rlocus : Gain
  Mux : Mux  Inputs=9
  Mux1 : Mux
  Scope : Scope
  Scope1 : Scope
  Sum : Sum  Inputs=|++
  Sum1 : Sum  Inputs=|++
  Sum4 : Sum  Inputs=|+-
  selector : Subsystem
  R(yaw) : Outport
  wires:
  Demux/7 -> Mux/7
  Demux/6 -> Mux/6
  Constant2/1 -> Integrator/2
  Demux/3 -> Mux/3
  Sum/1 -> Integrator/1
  selector/1(Out1) -> Scope1/1, KD_Based on Rlocus/1
  B/1 -> Demux/1
  Demux/2 -> Mux/2
  Demux/4 -> Mux/4
  Demux/9 -> Mux/9
  Integrator/1 -> selector/1(In1), Sum4/2, Scope/1, A/1
  Sum4/1 -> Sum/1
  A/1 -> Sum/2
  Demux/5 -> Mux/5
  Demux/1 -> Mux/1
  Mux/1 -> Sum4/1
  Mux1/1 -> B/1
  Constant1/1 -> Mux1/3, Mux1/2, Mux1/1
  Rudder/1 -> Mux1/4
  selector/2(Out2) -> R(yaw)/1
  Demux/8 -> Sum1/1
  KD_Based on Rlocus/1 -> Sum1/2
  Sum1/1 -> Mux/8

== system Perfect_Lineaer/Skid to turn (Lateral Dynamics don't change!)/Subsystem4 ==
  note: Inner loop
  note: State loop
  Rudder : Inport
  A : Gain  Gain=A  Multiplication=Matrix(K*u)
  B : Gain  Gain=B  Multiplication=Matrix(K*u)
  Constant1 : Constant  Value=0
  Constant2 : Constant  Value=X0
  Demux : Demux  Outputs=9
  Integrator : Integrator  InitialConditionSource=external
  KD_Based on Rlocus : Gain
  Mux : Mux  Inputs=9
  Mux1 : Mux
  Scope : Scope
  Scope1 : Scope
  Sum : Sum  Inputs=|++
  Sum1 : Sum  Inputs=|++
  Sum4 : Sum  Inputs=|+-
  selector : Subsystem
  R(yaw) : Outport
  wires:
  Demux/7 -> Mux/7
  Demux/6 -> Mux/6
  Constant2/1 -> Integrator/2
  Demux/3 -> Mux/3
  Sum/1 -> Integrator/1
  selector/1(Out1) -> Scope1/1, KD_Based on Rlocus/1
  B/1 -> Demux/1
  Demux/2 -> Mux/2
  Demux/4 -> Mux/4
  Demux/9 -> Mux/9
  Integrator/1 -> selector/1(In1), Sum4/2, Scope/1, A/1
  Sum4/1 -> Sum/1
  A/1 -> Sum/2
  Demux/5 -> Mux/5
  Demux/1 -> Mux/1
  Mux/1 -> Sum4/1
  Mux1/1 -> B/1
  Constant1/1 -> Mux1/3, Mux1/2, Mux1/1
  Rudder/1 -> Mux1/4
  selector/2(Out2) -> R(yaw)/1
  Demux/8 -> Sum1/1
  KD_Based on Rlocus/1 -> Sum1/2
  Sum1/1 -> Mux/8

== system Perfect_Lineaer/Skid to turn (Lateral Dynamics don't change!)/Subsystem5 ==
  note: Inner loop
  note: State loop
  Rudder : Inport
  Elevator : Inport  Port=2
  A : Gain  Gain=A  Multiplication=Matrix(K*u)
  B : Gain  Gain=B  Multiplication=Matrix(K*u)
  Constant1 : Constant  Value=0
  Constant2 : Constant  Value=X0
  Demux : Demux  Outputs=9
  Integrator : Integrator  InitialConditionSource=external
  KD_Based on Rlocus : Gain
  Mux : Mux  Inputs=9
  Mux1 : Mux
  Scope : Scope
  Scope1 : Scope
  Sum : Sum  Inputs=|++
  Sum1 : Sum  Inputs=|++
  Sum4 : Sum  Inputs=|+-
  selector : Subsystem
  R(yaw) : Outport
  Q(pitch) : Outport  Port=2
  wires:
  Demux/7 -> Mux/7
  Demux/6 -> Mux/6
  Constant2/1 -> Integrator/2
  Demux/3 -> Mux/3
  Sum/1 -> Integrator/1
  selector/1(Out1) -> Scope1/1, KD_Based on Rlocus/1
  B/1 -> Demux/1
  Demux/2 -> Mux/2
  Demux/4 -> Mux/4
  Demux/9 -> Mux/9
  Integrator/1 -> selector/1(In1), Sum4/2, Scope/1, A/1
  Sum4/1 -> Sum/1
  A/1 -> Sum/2
  Demux/5 -> Mux/5
  Demux/1 -> Mux/1
  Mux/1 -> Sum4/1
  Mux1/1 -> B/1
  Constant1/1 -> Mux1/2, Mux1/1
  Rudder/1 -> Mux1/4
  selector/2(yaw) -> R(yaw)/1
  Demux/8 -> Sum1/1
  KD_Based on Rlocus/1 -> Sum1/2
  Sum1/1 -> Mux/8
  selector/3(pitch) -> Q(pitch)/1
  Elevator/1 -> Mux1/3

== system Perfect_Lineaer/Skid to turn (Lateral Dynamics don't change!)/Subsystem6 ==
  note: Inner loop
  note: State loop
  Rudder : Inport
  A : Gain  Gain=A  Multiplication=Matrix(K*u)
  B : Gain  Gain=B  Multiplication=Matrix(K*u)
  Constant1 : Constant  Value=0
  Constant2 : Constant  Value=X0
  Demux : Demux  Outputs=9
  Integrator : Integrator  InitialConditionSource=external
  KD_Based on Rlocus : Gain
  Mux : Mux  Inputs=9
  Mux1 : Mux
  Scope : Scope
  Scope1 : Scope
  Sum : Sum  Inputs=|++
  Sum1 : Sum  Inputs=|++
  Sum4 : Sum  Inputs=|+-
  selector : Subsystem
  R(yaw) : Outport
  wires:
  Demux/7 -> Mux/7
  Demux/6 -> Mux/6
  Constant2/1 -> Integrator/2
  Demux/3 -> Mux/3
  Sum/1 -> Integrator/1
  selector/1(Out1) -> Scope1/1, KD_Based on Rlocus/1
  B/1 -> Demux/1
  Demux/2 -> Mux/2
  Demux/4 -> Mux/4
  Demux/9 -> Mux/9
  Integrator/1 -> selector/1(In1), Sum4/2, Scope/1, A/1
  Sum4/1 -> Sum/1
  A/1 -> Sum/2
  Demux/5 -> Mux/5
  Demux/1 -> Mux/1
  Mux/1 -> Sum4/1
  Mux1/1 -> B/1
  Constant1/1 -> Mux1/3, Mux1/2, Mux1/1
  Rudder/1 -> Mux1/4
  selector/2(Out2) -> R(yaw)/1
  Demux/8 -> Sum1/1
  KD_Based on Rlocus/1 -> Sum1/2
  Sum1/1 -> Mux/8

== system Perfect_Lineaer/Skid to turn (Lateral Dynamics don't change!)/Subsystem7 ==
  note: Inner loop
  note: State loop
  Aileron_r : Inport
  Aileron_l : Inport  Port=2
  A : Gain  Gain=A  Multiplication=Matrix(K*u)
  B : Gain  Gain=B  Multiplication=Matrix(K*u)
  Constant1 : Constant  Value=0
  Constant2 : Constant  Value=X0
  Demux : Demux  Outputs=9
  Integrator : Integrator  InitialConditionSource=external
  KD_Based on Rlocus : Gain
  Mux : Mux  Inputs=9
  Mux1 : Mux
  Scope : Scope
  Scope1 : Scope
  Sum : Sum  Inputs=|++
  Sum1 : Sum  Inputs=|++
  Sum4 : Sum  Inputs=|+-
  selector : Subsystem
  P(roll) : Outport
  wires:
  Demux/7 -> Mux/7
  Demux/6 -> Mux/6
  Constant2/1 -> Integrator/2
  Demux/3 -> Mux/3
  Sum/1 -> Integrator/1
  selector/1(Out1) -> Scope1/1, KD_Based on Rlocus/1
  B/1 -> Demux/1
  Demux/2 -> Mux/2
  Demux/4 -> Mux/4
  Demux/9 -> Mux/9
  Integrator/1 -> selector/1(In1), Sum4/2, Scope/1, A/1
  Sum4/1 -> Sum/1
  A/1 -> Sum/2
  Demux/5 -> Mux/5
  Demux/1 -> Mux/1
  Mux/1 -> Sum4/1
  Mux1/1 -> B/1
  Constant1/1 -> Mux1/3, Mux1/4
  selector/2(Out2) -> P(roll)/1
  Demux/8 -> Sum1/1
  KD_Based on Rlocus/1 -> Sum1/2
  Sum1/1 -> Mux/8
  Aileron_r/1 -> Mux1/1
  Aileron_l/1 -> Mux1/2

== system Perfect_Lineaer/Skid to turn (Lateral Dynamics don't change!)/Subsystem8 ==
  note: Inner loop
  note: State loop
  Aileron_r : Inport
  Aileron_l : Inport  Port=2
  A : Gain  Gain=A  Multiplication=Matrix(K*u)
  B : Gain  Gain=B  Multiplication=Matrix(K*u)
  Constant1 : Constant  Value=0
  Constant2 : Constant  Value=X0
  Demux : Demux  Outputs=9
  Integrator : Integrator  InitialConditionSource=external
  KD_Based on Rlocus : Gain
  Mux : Mux  Inputs=9
  Mux1 : Mux
  Scope : Scope
  Scope1 : Scope
  Sum : Sum  Inputs=|++
  Sum1 : Sum  Inputs=|++
  Sum4 : Sum  Inputs=|+-
  selector : Subsystem
  P(roll) : Outport
  wires:
  Demux/7 -> Mux/7
  Demux/6 -> Mux/6
  Constant2/1 -> Integrator/2
  Demux/3 -> Mux/3
  Sum/1 -> Integrator/1
  selector/1(Out1) -> Scope1/1, KD_Based on Rlocus/1
  B/1 -> Demux/1
  Demux/2 -> Mux/2
  Demux/4 -> Mux/4
  Demux/9 -> Mux/9
  Integrator/1 -> selector/1(In1), Sum4/2, Scope/1, A/1
  Sum4/1 -> Sum/1
  A/1 -> Sum/2
  Demux/5 -> Mux/5
  Demux/1 -> Mux/1
  Mux/1 -> Sum4/1
  Mux1/1 -> B/1
  Constant1/1 -> Mux1/3, Mux1/4
  selector/2(Out2) -> P(roll)/1
  Demux/8 -> Sum1/1
  KD_Based on Rlocus/1 -> Sum1/2
  Sum1/1 -> Mux/8
  Aileron_r/1 -> Mux1/1
  Aileron_l/1 -> Mux1/2

== system Perfect_Lineaer/Skid to turn (Lateral Dynamics don't change!)/Subsystem9 ==
  note: Inner loop
  note: State loop
  Aileron_r : Inport
  Aileron_l : Inport  Port=2
  A : Gain  Gain=A  Multiplication=Matrix(K*u)
  B : Gain  Gain=B  Multiplication=Matrix(K*u)
  Constant1 : Constant  Value=0
  Constant2 : Constant  Value=X0
  Demux : Demux  Outputs=9
  Integrator : Integrator  InitialConditionSource=external
  KD_Based on Rlocus : Gain
  Mux : Mux  Inputs=9
  Mux1 : Mux
  Scope : Scope
  Scope1 : Scope
  Sum : Sum  Inputs=|++
  Sum1 : Sum  Inputs=|++
  Sum4 : Sum  Inputs=|+-
  selector : Subsystem
  P(roll) : Outport
  wires:
  Demux/7 -> Mux/7
  Demux/6 -> Mux/6
  Constant2/1 -> Integrator/2
  Demux/3 -> Mux/3
  Sum/1 -> Integrator/1
  selector/1(Out1) -> Scope1/1, KD_Based on Rlocus/1
  B/1 -> Demux/1
  Demux/2 -> Mux/2
  Demux/4 -> Mux/4
  Demux/9 -> Mux/9
  Integrator/1 -> selector/1(In1), Sum4/2, Scope/1, A/1
  Sum4/1 -> Sum/1
  A/1 -> Sum/2
  Demux/5 -> Mux/5
  Demux/1 -> Mux/1
  Mux/1 -> Sum4/1
  Mux1/1 -> B/1
  Constant1/1 -> Mux1/3, Mux1/4
  selector/2(Out2) -> P(roll)/1
  Demux/8 -> Sum1/1
  KD_Based on Rlocus/1 -> Sum1/2
  Sum1/1 -> Mux/8
  Aileron_l/1 -> Mux1/2
  Aileron_r/1 -> Mux1/1

== system Perfect_Lineaer/Skid to turn (Lateral Dynamics)1/Subsystem ==
  note: Inner loop
  note: State loop
  Rudder : Inport
  A : Gain  Gain=A  Multiplication=Matrix(K*u)
  B : Gain  Gain=B  Multiplication=Matrix(K*u)
  Constant1 : Constant  Value=0
  Constant2 : Constant  Value=X0
  Demux : Demux  Outputs=9
  Integrator : Integrator  InitialConditionSource=external
  KD_Based on Rlocus : Gain
  Mux : Mux  Inputs=9
  Mux1 : Mux
  Scope : Scope
  Scope1 : Scope
  Sum : Sum  Inputs=|++
  Sum1 : Sum  Inputs=|++
  Sum4 : Sum  Inputs=|+-
  selector : Subsystem
  R(yaw) : Outport
  wires:
  Demux/7 -> Mux/7
  Demux/6 -> Mux/6
  Constant2/1 -> Integrator/2
  Demux/3 -> Mux/3
  Sum/1 -> Integrator/1
  selector/1(Out1) -> Scope1/1, KD_Based on Rlocus/1
  B/1 -> Demux/1
  Demux/2 -> Mux/2
  Demux/4 -> Mux/4
  Demux/9 -> Mux/9
  Integrator/1 -> selector/1(In1), Sum4/2, Scope/1, A/1
  Sum4/1 -> Sum/1
  A/1 -> Sum/2
  Demux/5 -> Mux/5
  Demux/1 -> Mux/1
  Mux/1 -> Sum4/1
  Mux1/1 -> B/1
  Constant1/1 -> Mux1/3, Mux1/2, Mux1/1
  Rudder/1 -> Mux1/4
  selector/2(Out2) -> R(yaw)/1
  Demux/8 -> Sum1/1
  KD_Based on Rlocus/1 -> Sum1/2
  Sum1/1 -> Mux/8

== system Perfect_Lineaer/Skid to turn (Lateral Dynamics)1/Subsystem1 ==
  note: Inner loop
  note: State loop
  Elevator : Inport
  A : Gain  Gain=A  Multiplication=Matrix(K*u)
  B : Gain  Gain=B  Multiplication=Matrix(K*u)
  Constant1 : Constant  Value=0
  Constant2 : Constant  Value=X0
  Demux : Demux  Outputs=9
  Integrator : Integrator  InitialConditionSource=external
  KD_Based on Rlocus : Gain
  Mux : Mux  Inputs=9
  Mux1 : Mux
  Scope : Scope
  Scope1 : Scope
  Sum : Sum  Inputs=|++
  Sum1 : Sum  Inputs=|++
  Sum4 : Sum  Inputs=|+-
  selector : Subsystem
  Q(pitch) : Outport
  wires:
  Demux/7 -> Mux/7
  Demux/6 -> Mux/6
  Constant2/1 -> Integrator/2
  Demux/3 -> Mux/3
  Sum/1 -> Integrator/1
  selector/1(Out1) -> Scope1/1, KD_Based on Rlocus/1
  B/1 -> Demux/1
  Demux/2 -> Mux/2
  Demux/4 -> Mux/4
  Demux/9 -> Mux/9
  Integrator/1 -> selector/1(In1), Sum4/2, Scope/1, A/1
  Sum4/1 -> Sum/1
  A/1 -> Sum/2
  Demux/5 -> Mux/5
  Demux/1 -> Mux/1
  Mux/1 -> Sum4/1
  Mux1/1 -> B/1
  Constant1/1 -> Mux1/2, Mux1/1, Mux1/4
  selector/2(Out2) -> Q(pitch)/1
  Demux/8 -> Sum1/1
  KD_Based on Rlocus/1 -> Sum1/2
  Sum1/1 -> Mux/8
  Elevator/1 -> Mux1/3

== system Perfect_Lineaer/Skid to turn (Lateral Dynamics)1/Subsystem2 ==
  note: Inner loop
  note: State loop
  Rudder : Inport
  A : Gain  Gain=A  Multiplication=Matrix(K*u)
  B : Gain  Gain=B  Multiplication=Matrix(K*u)
  Constant1 : Constant  Value=0
  Constant2 : Constant  Value=X0
  Demux : Demux  Outputs=9
  Integrator : Integrator  InitialConditionSource=external
  KD_Based on Rlocus : Gain
  Mux : Mux  Inputs=9
  Mux1 : Mux
  Scope : Scope
  Scope1 : Scope
  Sum : Sum  Inputs=|++
  Sum1 : Sum  Inputs=|++
  Sum4 : Sum  Inputs=|+-
  selector : Subsystem
  R(yaw) : Outport
  wires:
  Demux/7 -> Mux/7
  Demux/6 -> Mux/6
  Constant2/1 -> Integrator/2
  Demux/3 -> Mux/3
  Sum/1 -> Integrator/1
  selector/1(Out1) -> Scope1/1, KD_Based on Rlocus/1
  B/1 -> Demux/1
  Demux/2 -> Mux/2
  Demux/4 -> Mux/4
  Demux/9 -> Mux/9
  Integrator/1 -> selector/1(In1), Sum4/2, Scope/1, A/1
  Sum4/1 -> Sum/1
  A/1 -> Sum/2
  Demux/5 -> Mux/5
  Demux/1 -> Mux/1
  Mux/1 -> Sum4/1
  Mux1/1 -> B/1
  Constant1/1 -> Mux1/3, Mux1/2, Mux1/1
  Rudder/1 -> Mux1/4
  selector/2(Out2) -> R(yaw)/1
  Demux/8 -> Sum1/1
  KD_Based on Rlocus/1 -> Sum1/2
  Sum1/1 -> Mux/8
